simulink model "validate_throttle_request"  (R2015a)
settings: Solver=ode45  StartTime=0.0  StopTime=10.0  RelTol=1e-3
settings Model: Creator=Piyush  LastModifiedBy=Piyush

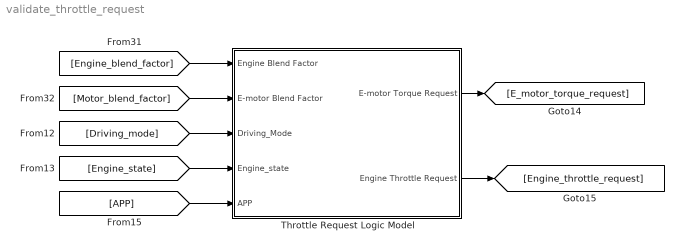
== system validate_throttle_request ==
  Throttle Request Logic Model : Subsystem
  wires:
  [Engine_blend_factor] -> Throttle Request Logic Model/1(Engine Blend Factor)
  [Motor_blend_factor] -> Throttle Request Logic Model/2(E-motor Blend Factor)
  [Driving_mode] -> Throttle Request Logic Model/3(Driving_Mode)
  [Engine_state] -> Throttle Request Logic Model/4(Engine_state)
  [APP] -> Throttle Request Logic Model/5(APP)
  Throttle Request Logic Model/1(E-motor Torque Request) -> [E_motor_torque_request]
  Throttle Request Logic Model/2(Engine Throttle Request) -> [Engine_throttle_request]

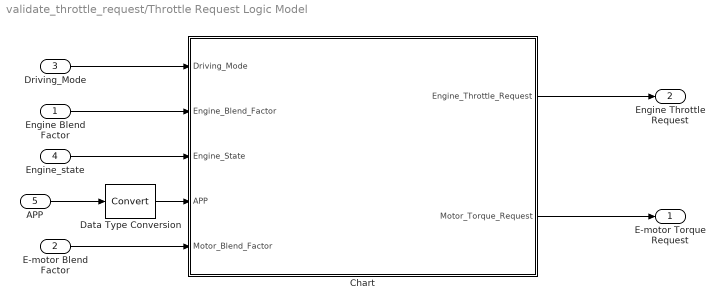
== system validate_throttle_request/Throttle Request Logic Model ==
  Engine Blend Factor : Inport
  E-motor Blend Factor : Inport  Port=2
  Driving_Mode : Inport  Port=3
  Engine_state : Inport  Port=4
  APP : Inport  Port=5
  Chart : Stateflow chart  TreatAsAtomicUnit=on
  Data Type Conversion : DataTypeConversion
  E-motor Torque Request : Outport
  Engine Throttle Request : Outport  Port=2
  wires:
  Engine Blend Factor/1 -> Chart/2(Engine_Blend_Factor)
  E-motor Blend Factor/1 -> Chart/5(Motor_Blend_Factor)
  APP/1 -> Data Type Conversion/1
  Engine_state/1 -> Chart/3(Engine_State)
  Driving_Mode/1 -> Chart/1(Driving_Mode)
  Chart/2(Motor_Torque_Request) -> E-motor Torque Request/1
  Chart/1(Engine_Throttle_Request) -> Engine Throttle Request/1
  Data Type Conversion/1 -> Chart/4(APP)

== stateflow chart validate_throttle_request/Throttle Request Logic Model/Chart ==
  state BlendingMode
    state State1
      during: Engine_Throttle_Request=7.5;
      during:Motor_Torque_Request=APP*Motor_Blend_Factor;
    state State2
      during: Engine_Throttle_Request=(APP*Engine_Blend_Factor);
      during: Motor_Torque_Request=APP*Motor_Blend_Factor;
    State2 -> State1 : [Engine_State==2||Engine_State==3]
    State1 -> State2 : [Engine_State==1||Engine_State==4||Engine_State==5]
    (default) -> State2
  state ElectricSoloMode
    during: Engine_Throttle_Request=0;
    during: Motor_Torque_Request=APP;
  state EngineSoloMode
    during:Engine_Throttle_Request=APP;
    during: Motor_Torque_Request = 0;
  (default) -> ElectricSoloMode
  ElectricSoloMode -> (junction 9) : [Driving_Mode==2||Driving_Mode==3]
  (junction 9) -> ElectricSoloMode [order 1] : [Driving_Mode==1]
  (junction 9) -> BlendingMode [order 2] : [Driving_Mode==2]
  (junction 9) -> EngineSoloMode [order 3] : [Driving_Mode==3]
  BlendingMode -> (junction 9) : [Driving_Mode==2||Driving_Mode==1]
  EngineSoloMode -> (junction 9) : [Driving_Mode==2||Driving_Mode==1]
  data: Driving_Mode input; Engine_Blend_Factor input; Engine_State input; APP input; Motor_Blend_Factor input; Engine_Throttle_Request output; Motor_Torque_Request output
